simulink model "WEC_Sim_Driver"  (R2013a)
settings: Solver=ode4  StartTime=StartTime  StopTime=EndTime  FixedStep=deltaT  MaxStep=deltaTMax  MinStep=deltaTMin  RelTol=1e-3
undefined symbols (not defined in the file): A_bore, A_c_F, A_c_P, A_rod, angle_arm_aft, Bd, C_aft, deltaT, Gen_Damp, hyd_mot_eff, hydro, hydroForce, Jtot, K_aft, Kd, mooring_c, mooring_k, nonlinear_params, omega_s, p_atm, p_hp, p_lp, pump_vol_eff, r_g, STLfloat, STLplate, Ts, V_hp, V_lp, Vg, X, Y, Z
libraries: nesl_utility x35, sm_lib x14
(part 1 of 2)
settings Model: Creator=cmccomb  LastModifiedBy=sakanne
settings SolverCC: InitialStep=deltaTInitial  MaxConsecutiveZCs=10000  MaxConsecutiveMinStep=20  ZeroCrossAlgorithm=Adaptive
settings DataIOCC: LimitDataPoints=off  SignalLoggingSaveFormat=ModelDataLogs
settings OptimizationCC: ExpressionDepthLimit=2147483647
settings DebuggingCC: FcnCallInpInsideContextMsg=EnableAllAsWarning

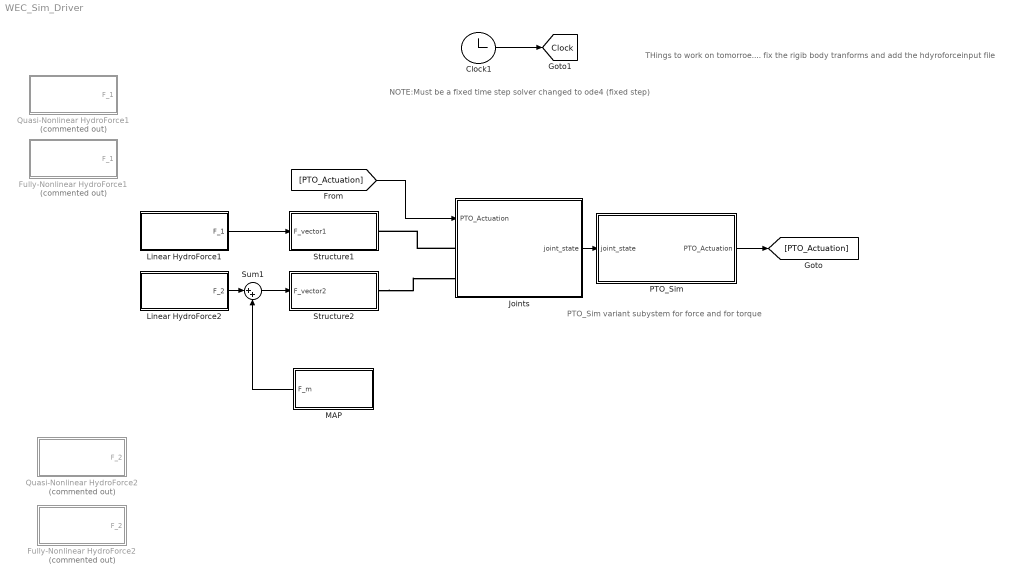
== system WEC_Sim_Driver ==
  note: THings to work on tomorroe....
      | fix the rigib body tranforms and add the hdyroforceinput file
  note: NOTE:Must be a fixed time step solver
      | changed to ode4 (fixed step)
  note: PTO_Sim variant subystem for force and for torque
  Clock1 : Clock
      settings: Decimation=50
  Fully-Nonlinear HydroForce1 : Subsystem  Commented=on  mask{K_mat=hydroForce.HGRes_1, Am_mat=hydroForce.Fadm_1, B_mat=hydroForce.Fdmp_1, X_mat=hydroForce.F_extTime_1}
      mask prompts: K_mat "Stiffness Matrix"; Am_mat "Added Mass Matrix"; B_mat "Radiation Damping Matrix"; X_mat "Excitation Matrix"
  Fully-Nonlinear HydroForce2 : Subsystem  Commented=on  mask{K_mat=hydroForce.HGRes_2, Am_mat=hydroForce.Fadm_2, B_mat=hydroForce.Fdmp_2, X_mat=hydroForce.F_extTime_2}
      mask prompts: K_mat "Stiffness Matrix"; Am_mat "Added Mass Matrix"; B_mat "Radiation Damping Matrix"; X_mat "Excitation Matrix"
  Joints : Subsystem  Variant=on
  Linear HydroForce1 : Subsystem  mask{K_mat=hydroForce.HGRes_1, Am_mat=hydroForce.Fadm_1, B_mat=hydroForce.Fdmp_1, X_mat=hydroForce.F_extTime_1}
      mask prompts: K_mat "Stiffness Matrix"; Am_mat "Added Mass Matrix"; B_mat "Radiation Damping Matrix"; X_mat "Excitation Matrix"
  Linear HydroForce2 : Subsystem  mask{K_mat=hydroForce.HGRes_2, Am_mat=hydroForce.Fadm_2, B_mat=hydroForce.Fdmp_2, X_mat=hydroForce.F_extTime_2}
      mask prompts: K_mat "Stiffness Matrix"; Am_mat "Added Mass Matrix"; B_mat "Radiation Damping Matrix"; X_mat "Excitation Matrix"
  MAP : Subsystem
  PTO_Sim : Subsystem
  Quasi-Nonlinear HydroForce1 : Subsystem  Commented=on  mask{K_mat=hydroForce.HGRes_1, Am_mat=hydroForce.Fadm_1, B_mat=hydroForce.Fdmp_1, X_mat=hydroForce.F_extTime_1}
      mask prompts: K_mat "Stiffness Matrix"; Am_mat "Added Mass Matrix"; B_mat "Radiation Damping Matrix"; X_mat "Excitation Matrix"
  Quasi-Nonlinear HydroForce2 : Subsystem  Commented=on  mask{K_mat=hydroForce.HGRes_2, Am_mat=hydroForce.Fadm_2, B_mat=hydroForce.Fdmp_2, X_mat=hydroForce.F_extTime_2}
      mask prompts: K_mat "Stiffness Matrix"; Am_mat "Added Mass Matrix"; B_mat "Radiation Damping Matrix"; X_mat "Excitation Matrix"
  Structure1 : Subsystem
  Structure2 : Subsystem
  Sum1 : Sum  Inputs=|++
  tag scope: Clock=global
  wires:
  Joints/1(joint_state) -> PTO_Sim/1(joint_state)
  MAP/1(F_m) -> Sum1/2
  PTO_Sim/1(PTO_Actuation) -> [PTO_Actuation]
  [PTO_Actuation] -> Joints/1(PTO_Actuation)
  Sum1/1 -> Structure2/1(F_vector2)
  Clock1/1 -> [Clock]
  Linear HydroForce2/1(F_2) -> Sum1/1
  Linear HydroForce1/1(F_1) -> Structure1/1(F_vector1)
  connections:
  Joints/LConn1 -- Structure1/RConn1
  Structure2/RConn1 -- Joints/LConn2

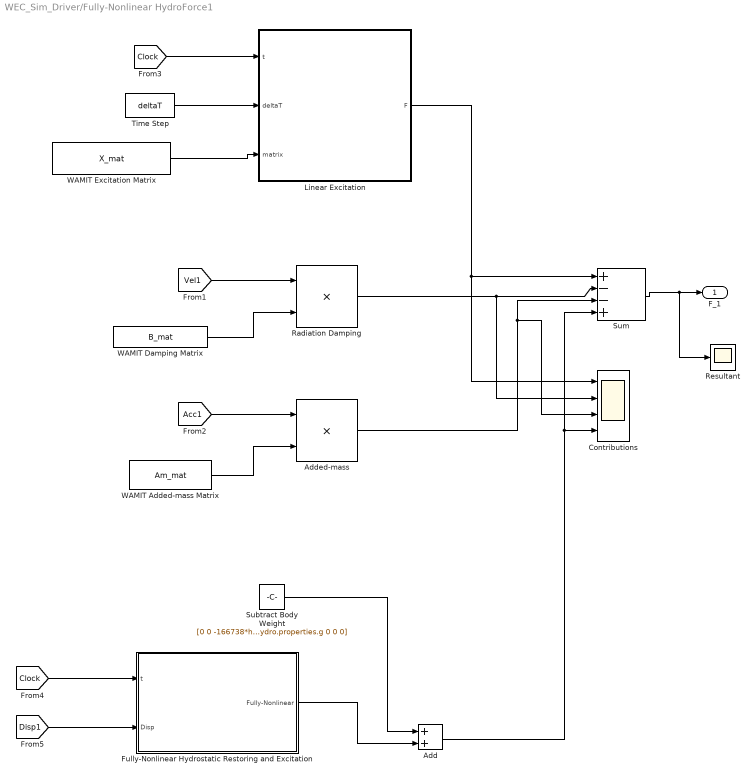
== system WEC_Sim_Driver/Fully-Nonlinear HydroForce1 ==
  Add : Sum
  Added-mass : Product
  Contributions : Scope  NumInputPorts=4
      settings: YMin=-5~-5~-5~-5  YMax=5~5~5~5  SaveName=ScopeData2
  Fully-Nonlinear Hydrostatic Restoring and Excitation : Subsystem  TreatAsAtomicUnit=on
  Linear Excitation : MATLAB Function  TreatAsAtomicUnit=on
  Radiation Damping : Product
  Resultant : Scope
  Subtract Body Weight : Constant  Value=[0 0 -166738*hydro.properties.g 0 0 0]
  Sum : Sum  Inputs=+--+
  Time Step : Constant  Value=deltaT
  WAMIT Added-mass Matrix : Constant  Value=Am_mat  VectorParams1D=off
  WAMIT Damping Matrix : Constant  Value=B_mat  VectorParams1D=off
  WAMIT Excitation Matrix : Constant  Value=X_mat  VectorParams1D=off
  F_1 : Outport
  wires:
  Radiation Damping/1 -> Sum/2, Contributions/2
  [Vel1] -> Radiation Damping/1
  WAMIT Damping Matrix/1 -> Radiation Damping/2
  Added-mass/1 -> Sum/3, Contributions/3
  [Acc1] -> Added-mass/1
  WAMIT Added-mass Matrix/1 -> Added-mass/2
  Sum/1 -> Resultant/1, F_1/1
  [Clock] -> Fully-Nonlinear Hydrostatic Restoring and Excitation/1(t)
  [Disp1] -> Fully-Nonlinear Hydrostatic Restoring and Excitation/2(Disp)
  Subtract Body Weight/1 -> Add/1
  Fully-Nonlinear Hydrostatic Restoring and Excitation/1(Fully-Nonlinear) -> Add/2
  Time Step/1 -> Linear Excitation/2(deltaT)
  WAMIT Excitation Matrix/1 -> Linear Excitation/3(matrix)
  [Clock] -> Linear Excitation/1(t)
  Linear Excitation/1(F) -> Sum/1, Contributions/1
  Add/1 -> Contributions/4, Sum/4

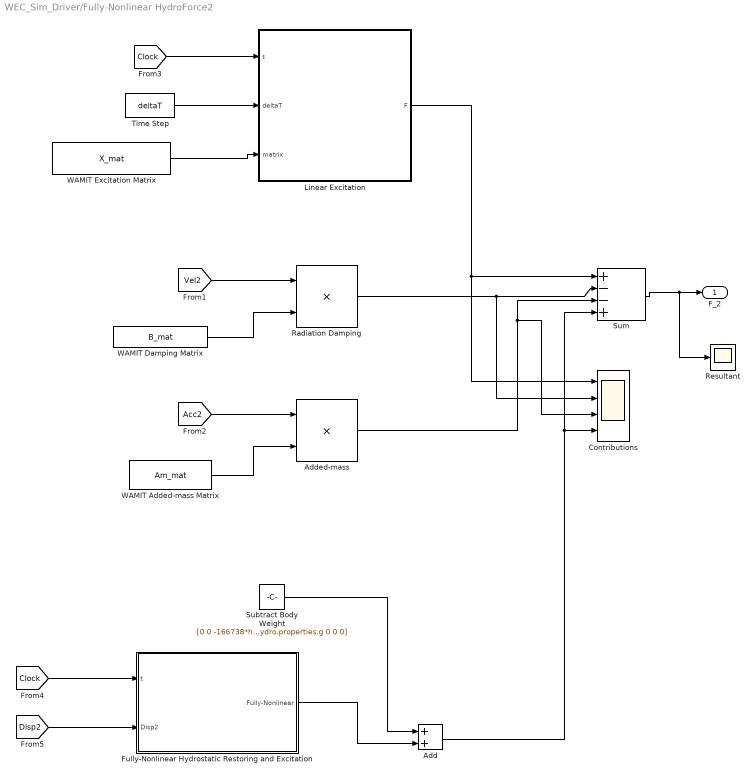
== system WEC_Sim_Driver/Fully-Nonlinear HydroForce2 ==
  Add : Sum
  Added-mass : Product
  Contributions : Scope  NumInputPorts=4
      settings: YMin=-5~-5~-5~-5  YMax=5~5~5~5  SaveName=ScopeData2
  Fully-Nonlinear Hydrostatic Restoring and Excitation : Subsystem  TreatAsAtomicUnit=on
  Linear Excitation : MATLAB Function  TreatAsAtomicUnit=on
  Radiation Damping : Product
  Resultant : Scope
  Subtract Body Weight : Constant  Value=[0 0 -166738*hydro.properties.g 0 0 0]
  Sum : Sum  Inputs=+--+
  Time Step : Constant  Value=deltaT
  WAMIT Added-mass Matrix : Constant  Value=Am_mat  VectorParams1D=off
  WAMIT Damping Matrix : Constant  Value=B_mat  VectorParams1D=off
  WAMIT Excitation Matrix : Constant  Value=X_mat  VectorParams1D=off
  F_2 : Outport
  wires:
  Radiation Damping/1 -> Sum/2, Contributions/2
  [Vel2] -> Radiation Damping/1
  WAMIT Damping Matrix/1 -> Radiation Damping/2
  Added-mass/1 -> Sum/3, Contributions/3
  [Acc2] -> Added-mass/1
  WAMIT Added-mass Matrix/1 -> Added-mass/2
  Sum/1 -> Resultant/1, F_2/1
  [Clock] -> Fully-Nonlinear Hydrostatic Restoring and Excitation/1(t)
  [Disp2] -> Fully-Nonlinear Hydrostatic Restoring and Excitation/2(Disp2)
  Subtract Body Weight/1 -> Add/1
  Fully-Nonlinear Hydrostatic Restoring and Excitation/1(Fully-Nonlinear) -> Add/2
  Time Step/1 -> Linear Excitation/2(deltaT)
  WAMIT Excitation Matrix/1 -> Linear Excitation/3(matrix)
  [Clock] -> Linear Excitation/1(t)
  Linear Excitation/1(F) -> Sum/1, Contributions/1
  Add/1 -> Contributions/4, Sum/4

== system WEC_Sim_Driver/Joints ==
  note: If you have a rotaional joint, you're outputing a torque and must change PTO-Sim to torque model.
      | similar is true to a linear joint and PTO
  note: 1) Only subsystems can be added as variant choices at this level
      | 2) Blocks cannot be connected at this level as connectivity is
      | automatically determined at simulation, based on the active variant
  PTO_Actuation : Inport
  Linear  Joint : Subsystem  VariantControl=VSS_Linear
  Rotational Joint : Subsystem  VariantControl=VSS_Rotation
  Body1 : PMIOPort  Port=1  Side=Left
  Body2 : PMIOPort  Port=2  Side=Left
  joint_state : Outport

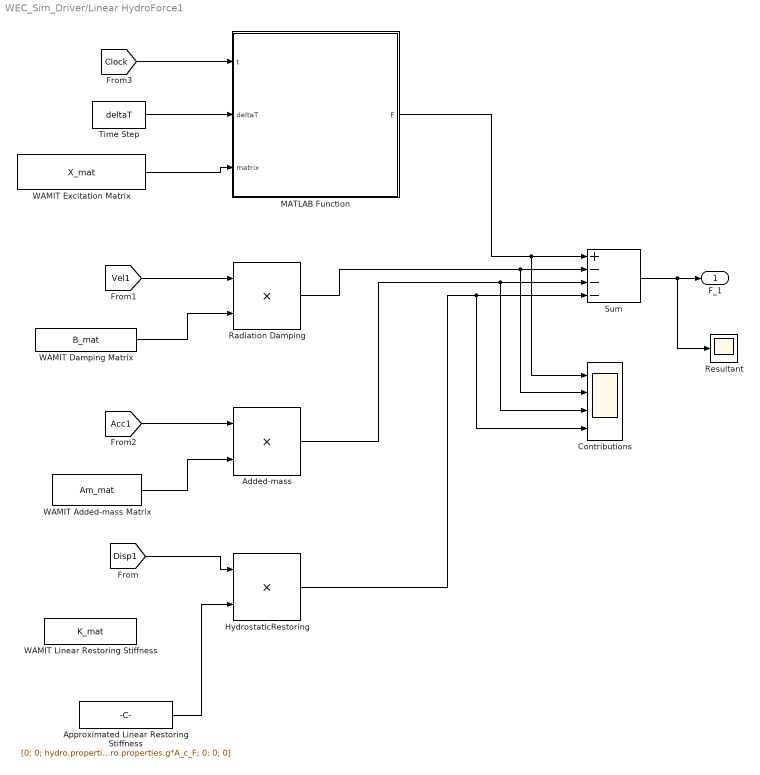
== system WEC_Sim_Driver/Linear HydroForce1 ==
  Added-mass : Product
  Approximated Linear Restoring Stiffness : Constant  Value=[0; 0; hydro.properties.density*hydro.properties.g*A_c_F; 0; 0; 0]  VectorParams1D=off
  Contributions : Scope  NumInputPorts=4
      settings: YMin=-5~-5~-5~-5  YMax=5~5~5~5  SaveName=ScopeData5
  HydrostaticRestoring : Product
  MATLAB Function : MATLAB Function  TreatAsAtomicUnit=on
  Radiation Damping : Product
  Resultant : Scope
      settings: SaveName=ScopeData6
  Sum : Sum  Inputs=+---
  Time Step : Constant  Value=deltaT
  WAMIT Added-mass Matrix : Constant  Value=Am_mat  VectorParams1D=off
  WAMIT Damping Matrix : Constant  Value=B_mat  VectorParams1D=off
  WAMIT Excitation Matrix : Constant  Value=X_mat  VectorParams1D=off
  WAMIT Linear Restoring Stiffness : Constant  Value=K_mat  VectorParams1D=off
  F_1 : Outport
  wires:
  Time Step/1 -> MATLAB Function/2(deltaT)
  WAMIT Excitation Matrix/1 -> MATLAB Function/3(matrix)
  MATLAB Function/1(F) -> Contributions/1, Sum/1
  Sum/1 -> F_1/1, Resultant/1
  WAMIT Added-mass Matrix/1 -> Added-mass/2
  [Acc1] -> Added-mass/1
  Added-mass/1 -> Contributions/3, Sum/3
  [Disp1] -> HydrostaticRestoring/1
  HydrostaticRestoring/1 -> Contributions/4, Sum/4
  WAMIT Damping Matrix/1 -> Radiation Damping/2
  [Vel1] -> Radiation Damping/1
  Radiation Damping/1 -> Contributions/2, Sum/2
  [Clock] -> MATLAB Function/1(t)
  Approximated Linear Restoring Stiffness/1 -> HydrostaticRestoring/2

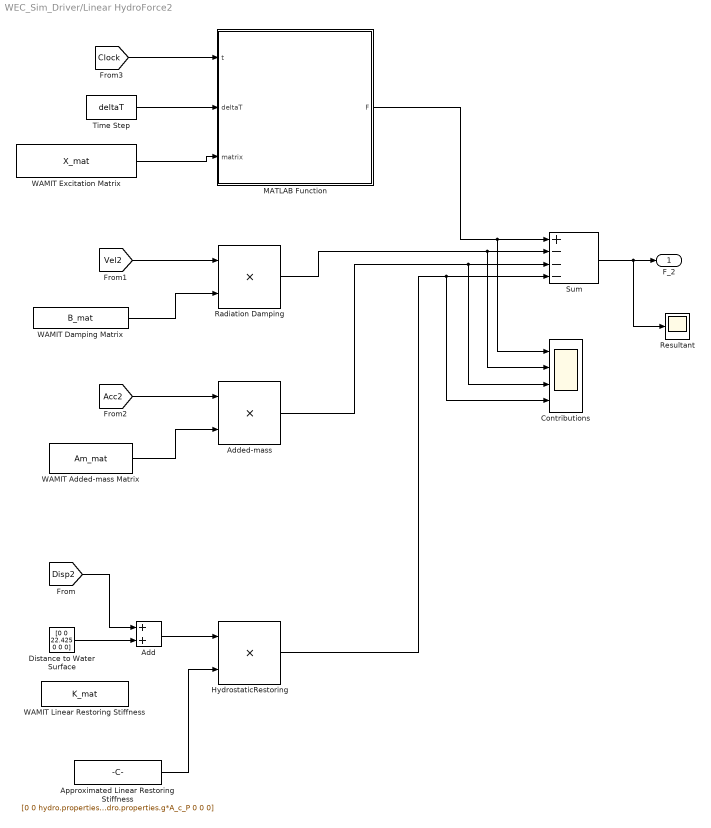
== system WEC_Sim_Driver/Linear HydroForce2 ==
  Add : Sum
  Added-mass : Product
  Approximated Linear Restoring Stiffness : Constant  Value=[0 0 hydro.properties.density*hydro.properties.g*A_c_P 0 0 0]  VectorParams1D=off
  Contributions : Scope  NumInputPorts=4
      settings: YMin=-5~-5~-5~-5  YMax=5~5~5~5  SaveName=ScopeData5
  Distance to Water Surface : Constant  Value=[0 0 22.425 0 0 0]
  HydrostaticRestoring : Product
  MATLAB Function : MATLAB Function  TreatAsAtomicUnit=on
  Radiation Damping : Product
  Resultant : Scope
      settings: SaveName=ScopeData6
  Sum : Sum  Inputs=+---
  Time Step : Constant  Value=deltaT
  WAMIT Added-mass Matrix : Constant  Value=Am_mat  VectorParams1D=off
  WAMIT Damping Matrix : Constant  Value=B_mat  VectorParams1D=off
  WAMIT Excitation Matrix : Constant  Value=X_mat  VectorParams1D=off
  WAMIT Linear Restoring Stiffness : Constant  Value=K_mat  VectorParams1D=off
  F_2 : Outport
  wires:
  Time Step/1 -> MATLAB Function/2(deltaT)
  WAMIT Excitation Matrix/1 -> MATLAB Function/3(matrix)
  MATLAB Function/1(F) -> Contributions/1, Sum/1
  Sum/1 -> F_2/1, Resultant/1
  WAMIT Added-mass Matrix/1 -> Added-mass/2
  [Acc2] -> Added-mass/1
  Added-mass/1 -> Contributions/3, Sum/3
  HydrostaticRestoring/1 -> Contributions/4, Sum/4
  WAMIT Damping Matrix/1 -> Radiation Damping/2
  [Vel2] -> Radiation Damping/1
  Radiation Damping/1 -> Contributions/2, Sum/2
  [Clock] -> MATLAB Function/1(t)
  Approximated Linear Restoring Stiffness/1 -> HydrostaticRestoring/2
  [Disp2] -> Add/1
  Add/1 -> HydrostaticRestoring/1
  Distance to Water Surface/1 -> Add/2

== system WEC_Sim_Driver/MAP ==
  Mooring damping : Gain  Gain=mooring_c  Multiplication=Matrix(K*u)
  Mooring stifness : Gain  Gain=mooring_k  Multiplication=Matrix(K*u)
  sum : Sum  Inputs=--
  F_m : Outport
  wires:
  Mooring stifness/1 -> sum/1
  Mooring damping/1 -> sum/2
  sum/1 -> F_m/1
  [Disp2] -> Mooring stifness/1
  [Vel2] -> Mooring damping/1

== system WEC_Sim_Driver/PTO_Sim ==
  joint_state : Inport
  Drivetrain : Subsystem  Variant=on  VariantControl=Variant
  Electricity_Generation : Subsystem  Variant=on  VariantControl=Variant1
  PTO_Actuation : Outport
  wires:
  Drivetrain/2(omega_Gen) -> Electricity_Generation/1(omega_gen_in)
  Electricity_Generation/1(T_gen_out) -> Drivetrain/2(T_gens_toDrivetrain)
  joint_state/1 -> Drivetrain/1(states_to_Drivetrain)
  Drivetrain/1(T_gen_out) -> PTO_Actuation/1

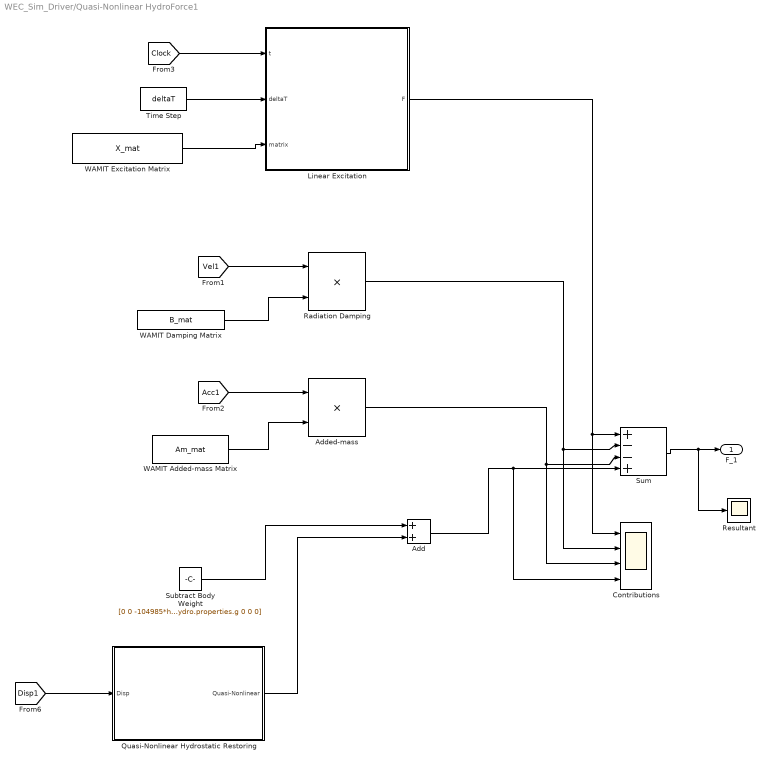
== system WEC_Sim_Driver/Quasi-Nonlinear HydroForce1 ==
  Add : Sum
  Added-mass : Product
  Contributions : Scope  NumInputPorts=4
      settings: YMin=-250000~-900~-35000~-60000  YMax=400000~50~55000~5000  SaveName=ScopeData2
  Linear Excitation : MATLAB Function  TreatAsAtomicUnit=on
  Quasi-Nonlinear Hydrostatic Restoring : Subsystem  TreatAsAtomicUnit=on
  Radiation Damping : Product
  Resultant : Scope
  Subtract Body Weight : Constant  Value=[0 0 -104985*hydro.properties.g 0 0 0]
  Sum : Sum  Inputs=+--+
  Time Step : Constant  Value=deltaT
  WAMIT Added-mass Matrix : Constant  Value=Am_mat  VectorParams1D=off
  WAMIT Damping Matrix : Constant  Value=B_mat  VectorParams1D=off
  WAMIT Excitation Matrix : Constant  Value=X_mat  VectorParams1D=off
  F_1 : Outport
  wires:
  Subtract Body Weight/1 -> Add/1
  Quasi-Nonlinear Hydrostatic Restoring/1(Quasi-Nonlinear) -> Add/2
  Time Step/1 -> Linear Excitation/2(deltaT)
  WAMIT Excitation Matrix/1 -> Linear Excitation/3(matrix)
  [Clock] -> Linear Excitation/1(t)
  [Disp1] -> Quasi-Nonlinear Hydrostatic Restoring/1(Disp)
  Sum/1 -> F_1/1, Resultant/1
  WAMIT Added-mass Matrix/1 -> Added-mass/2
  [Acc1] -> Added-mass/1
  Added-mass/1 -> Contributions/3, Sum/3
  WAMIT Damping Matrix/1 -> Radiation Damping/2
  [Vel1] -> Radiation Damping/1
  Radiation Damping/1 -> Contributions/2, Sum/2
  Linear Excitation/1(F) -> Contributions/1, Sum/1
  Add/1 -> Contributions/4, Sum/4

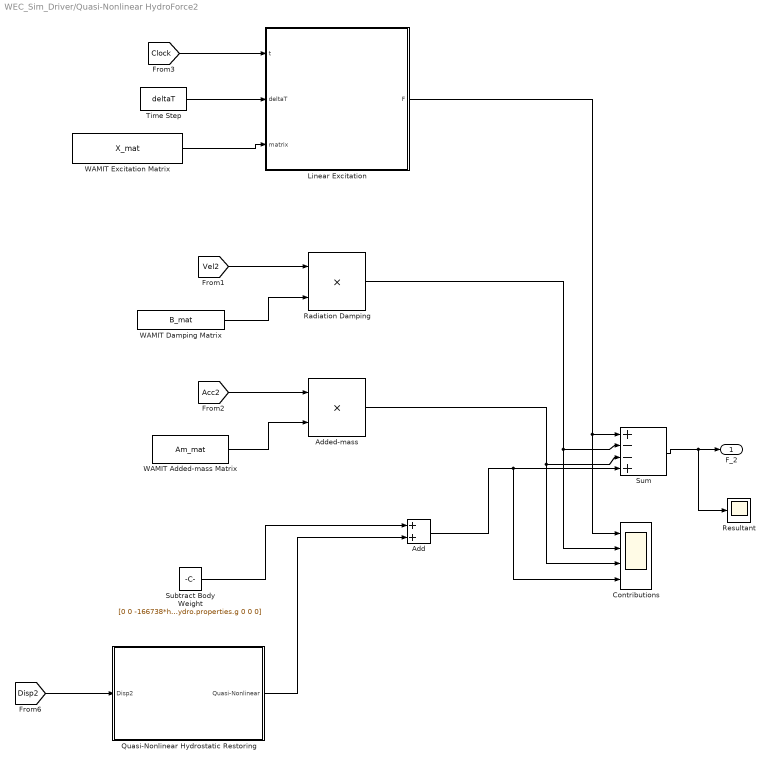
== system WEC_Sim_Driver/Quasi-Nonlinear HydroForce2 ==
  Add : Sum
  Added-mass : Product
  Contributions : Scope  NumInputPorts=4
      settings: YMin=-250000~-900~-35000~-60000  YMax=400000~50~55000~5000  SaveName=ScopeData2
  Linear Excitation : MATLAB Function  TreatAsAtomicUnit=on
  Quasi-Nonlinear Hydrostatic Restoring : Subsystem  TreatAsAtomicUnit=on
  Radiation Damping : Product
  Resultant : Scope
  Subtract Body Weight : Constant  Value=[0 0 -166738*hydro.properties.g 0 0 0]
  Sum : Sum  Inputs=+--+
  Time Step : Constant  Value=deltaT
  WAMIT Added-mass Matrix : Constant  Value=Am_mat  VectorParams1D=off
  WAMIT Damping Matrix : Constant  Value=B_mat  VectorParams1D=off
  WAMIT Excitation Matrix : Constant  Value=X_mat  VectorParams1D=off
  F_2 : Outport
  wires:
  Subtract Body Weight/1 -> Add/1
  Quasi-Nonlinear Hydrostatic Restoring/1(Quasi-Nonlinear) -> Add/2
  Time Step/1 -> Linear Excitation/2(deltaT)
  WAMIT Excitation Matrix/1 -> Linear Excitation/3(matrix)
  [Clock] -> Linear Excitation/1(t)
  [Disp2] -> Quasi-Nonlinear Hydrostatic Restoring/1(Disp2)
  Sum/1 -> F_2/1, Resultant/1
  WAMIT Added-mass Matrix/1 -> Added-mass/2
  [Acc2] -> Added-mass/1
  Added-mass/1 -> Contributions/3, Sum/3
  WAMIT Damping Matrix/1 -> Radiation Damping/2
  [Vel2] -> Radiation Damping/1
  Radiation Damping/1 -> Contributions/2, Sum/2
  Linear Excitation/1(F) -> Contributions/1, Sum/1
  Add/1 -> Contributions/4, Sum/4

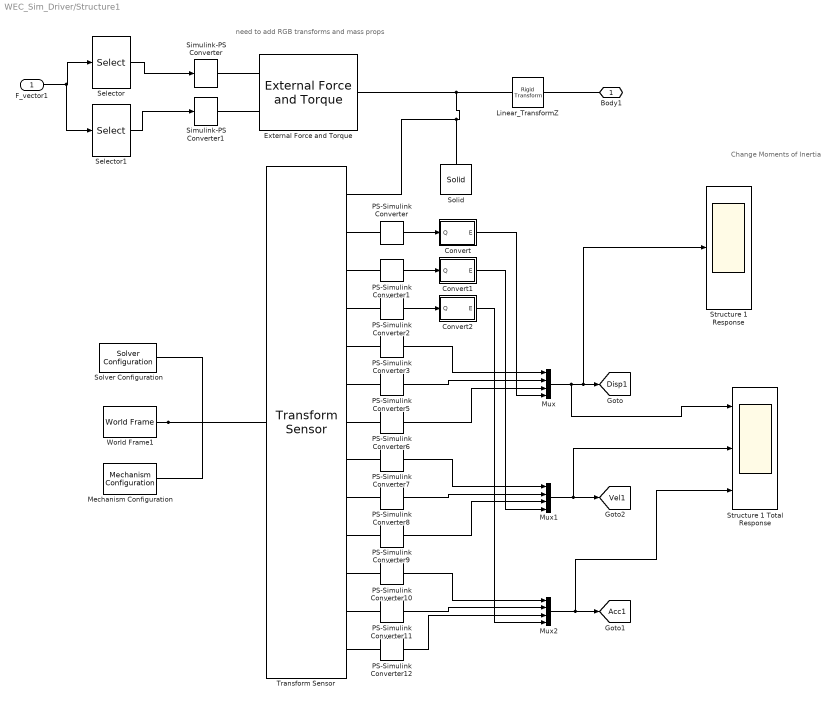
== system WEC_Sim_Driver/Structure1 ==
  note: Change Moments of Inertia
  note: need to add RGB transforms and mass props
  F_vector1 : Inport
  Convert : MATLAB Function  TreatAsAtomicUnit=on
  Convert1 : MATLAB Function  TreatAsAtomicUnit=on
  Convert2 : MATLAB Function  TreatAsAtomicUnit=on
  External Force and Torque : sm_lib/Forces and  Torques/External Force  and Torque  ForceResolutionFrame=AttachedFrame  EnableForceX=off  EnableForceY=off  EnableForceZ=off  EnableForce=on  TorqueResolutionFrame=AttachedFrame  EnableTorqueX=off  EnableTorqueY=off  EnableTorqueZ=off  EnableTorque=on  BlockFunction=simmechanics.library.forces_torques.external_force_torque
  Linear_TransformZ : sm_lib/Frames and  Transforms/Rigid  Transform  TranslationMethod=Cartesian  TranslationLengthUnit=m  TranslationStandardAxis=+Z  TranslationStandardOffset=0  TranslationCartesianOffset=[0 0 -22.425]  TranslationROffset=0  TranslationROffsetUnits=m  TranslationZOffset=0  TranslationZOffsetUnits=m  TranslationThetaOffset=0  TranslationThetaOffsetUnits=deg  RotationMethod=None  RotationAngleUnits=rad  RotationStandardAxis=+Z  RotationAngle=2.0943951023931953  RotationArbitraryAxis=[0.57735026918962584 0.57735026918962584 0.57735026918962584]  FollAlignAxisA=+X  BaseAlignAxisA=+Y  FollAlignAxisB=+Y  BaseAlignAxisB=+Z  BlockFunction=simmechanics.library.frames_transforms.rigid_transform
  Mechanism Configuration : sm_lib/Utilities/Mechanism  Configuration  GravityVector=[0 0 0]  GravityUnits=m/s^2  AllowGravitySignal=off  LinearizationDelta=0.001  BlockFunction=simmechanics.library.utilities.mechanism_configuration
  Mux : Mux
  Mux1 : Mux
  Mux2 : Mux
  PS-Simulink Converter{,1..3,5..12} (12 alike) : nesl_utility/PS-Simulink Converter  PhysicalDomain=network_engine_domain  SubClassName=ps_output  LeftPortType=input  RightPortType=output  PseudoPeriodic=off  Frequencies=[]  Unit=1  AffineConversion=off
  Selector : Selector  InputPortWidth=6  IndexOptions=Index vector (dialog)  Indices=[1:3]  OutputSizes=1
  Selector1 : Selector  InputPortWidth=6  IndexOptions=Index vector (dialog)  Indices=[4:6]  OutputSizes=1
  Simulink-PS Converter : nesl_utility/Simulink-PS Converter  PhysicalDomain=network_engine_domain  SubClassName=ps_input  LeftPortType=input  RightPortType=output  PseudoPeriodic=off  Frequencies=[]  NoiseDistribution=none  NoiseParameters=[]  Unit=1  AffineConversion=off  InputFiltering=off  SimscapeFilterOrder=1  InputFilterTimeConstant=0.001  UdotUserProvided=1
  Simulink-PS Converter1 : nesl_utility/Simulink-PS Converter  PhysicalDomain=network_engine_domain  SubClassName=ps_input  LeftPortType=input  RightPortType=output  PseudoPeriodic=off  Frequencies=[]  NoiseDistribution=none  NoiseParameters=[]  Unit=1  AffineConversion=off  InputFiltering=off  SimscapeFilterOrder=1  InputFilterTimeConstant=0.001  UdotUserProvided=1
  Solid : sm_lib/Body Elements/Solid  InertiaType=Custom  Mass=746000  MassUnits=kg  CenterOfMass=[0 0 0]  CenterOfMassUnits=m  MomentsOfInertia=[913451 913451 1704302]  MomentsOfInertiaUnits=kg*m^2  ProductsOfInertia=[0 0 0]  ProductsOfInertiaUnits=kg*m^2  DensityBased=on  Density=1000  DensityUnits=kg/(m^3)  GraphicType=FromGeometry  MarkerShape=Sphere  MarkerSize=10  MarkerSizeUnits=m  GraphicVisPropType=SimpleVisualProperties  GraphicDiffuseColor=[1 1 1]  GraphicSpecularColor=[0.5 0.5 0.5 1.0]  GraphicAmbientColor=[0.15 0.15 0.15 1.0]  GraphicEmissiveColor=[0.0 0.0 0.0 1.0]  GraphicShininess=75  GraphicOpacity=1  GeometryShape=FromFile  RectangleSize=[1 1]  RectangleSizeUnits=m  BrickDimensions=[1 1 1]  BrickDimensionUnits=m  CylinderRadius=1  CylinderRadiusUnits=m  CylinderLength=1  CylinderLengthUnits=m  SphereRadius=1  SphereRadiusUnits=m  EllipsoidRadii=[1 1 1]  EllipsoidRadiiUnits=m  ExtrusionCrossSection=[1 1; -1 1; -1 -1; 1 -1]  ExtrusionCrossSectionUnits=m  ExtrusionLength=1  ExtrusionLengthUnits=m  PolygonNumSides=3  PolygonOuterRadius=1  PolygonOuterRadiusUnits=m  ExtGeomFileName=\user_inputs\geometry\Float.STL  ExtGeomFileUnits=m  RevolutionCrossSection=[1 1; 1 -1; 2 -1; 2 1]  RevolutionCrossSectionUnits=m  RevolutionExtent=Full  RevolutionAngle=180  RevolutionAngleUnits=deg  BlockFunction=simmechanics.library.body_elements.solid
  Solver Configuration : nesl_utility/Solver Configuration  PhysicalDomain=network_engine_domain  SubClassName=solver  LeftPortType=input  RightPortType=generic  Accelerate=off  Tones=[]  Harmonics=[]  SimulateNoise=off  Profile=off  UseLocalSampling=off  EnableSwitchedLinearOptims=on  FrequencyDomain=off  UseCCode=off  UseNewInitialization=off  DoDC=on  ResidualTolerance=1e-9  UseLocalSolver=off  LocalSolverChoice=NE_BACKWARD_EULER_ADVANCER  LocalSolverSampleTime=.001  DoFixedCost=off  MaxNonlinIter=3  MaxModeIter=2  LinearAlgebra=Sparse  DelaysMemoryBudget=1024
  Structure 1 Response : Scope
      settings: ShowLegends=on  YMin=-1  YMax=1  SaveName=Structure1Response
  Structure 1 Total Response : Scope  NumInputPorts=3
      settings: ShowLegends=on  YMin=-1.5~-0.8~-0.5  YMax=1.5~0.8~0.5  SaveName=ScopeData3
  Transform Sensor : sm_lib/Frames and  Transforms/Transform  Sensor  MeasurementFrame=World  SenseAngle=off  SenseAxis=off  SenseAngle1=off  SenseAngle2=off  SenseAngle3=off  SenseQ=on  SenseR=off  SenseOmegaX=off  SenseOmegaY=off  SenseOmegaZ=off  SenseOmega1=off  SenseOmega2=off  SenseOmega3=off  SenseQDot=on  SenseRDot=off  SenseAlphaX=off  SenseAlphaY=off  SenseAlphaZ=off  SenseAlpha1=off  SenseAlpha2=off  SenseAlpha3=off  SenseQDDot=on  SenseRDDot=off  SenseX=on  SenseY=on  SenseZ=on  SenseRad=off  SenseAzim=off  SenseDist=off  SenseInc=off  SenseXDot=on  SenseYDot=on  SenseZDot=on  SenseRadDot=off  SenseAzimDot=off  SenseDistDot=off  SenseIncDot=off  SenseXDDot=on  SenseYDDot=on  SenseZDDot=on  SenseRadDDot=off  SenseAzimDDot=off  SenseDistDDot=off  SenseIncDDot=off  BlockFunction=simmechanics.library.frames_transforms.transform_sensor
  World Frame1 : sm_lib/Frames and  Transforms/World Frame  BlockFunction=simmechanics.library.frames_transforms.world_frame
  Body1 : PMIOPort  Port=1  Side=Right
  tag scope: Acc1=global, Disp1=global, Vel1=global
  wires:
  Mux/1 -> Structure 1 Total Response/1, Structure 1 Response/1, [Disp1]
  Mux1/1 -> Structure 1 Total Response/2, [Vel1]
  Mux2/1 -> Structure 1 Total Response/3, [Acc1]
  F_vector1/1 -> Selector1/1, Selector/1
  Selector/1 -> Simulink-PS Converter/1
  Selector1/1 -> Simulink-PS Converter1/1
  PS-Simulink Converter2/1 -> Convert2/1(Q)
  PS-Simulink Converter1/1 -> Convert1/1(Q)
  PS-Simulink Converter/1 -> Convert/1(Q)
  Convert/1(E) -> Mux/4
  Convert1/1(E) -> Mux1/4
  Convert2/1(E) -> Mux2/4
  PS-Simulink Converter3/1 -> Mux/1
  PS-Simulink Converter5/1 -> Mux/2
  PS-Simulink Converter6/1 -> Mux/3
  PS-Simulink Converter7/1 -> Mux1/1
  PS-Simulink Converter8/1 -> Mux1/2
  PS-Simulink Converter9/1 -> Mux1/3
  PS-Simulink Converter10/1 -> Mux2/1
  PS-Simulink Converter11/1 -> Mux2/2
  PS-Simulink Converter12/1 -> Mux2/3
  connections:
  Transform Sensor/RConn2 -- PS-Simulink Converter/LConn1
  PS-Simulink Converter1/LConn1 -- Transform Sensor/RConn3
  PS-Simulink Converter2/LConn1 -- Transform Sensor/RConn4
  PS-Simulink Converter3/LConn1 -- Transform Sensor/RConn5
  Transform Sensor/RConn12 -- PS-Simulink Converter11/LConn1
  Transform Sensor/RConn13 -- PS-Simulink Converter12/LConn1
  Transform Sensor/RConn10 -- PS-Simulink Converter9/LConn1
  Transform Sensor/RConn11 -- PS-Simulink Converter10/LConn1
  Transform Sensor/RConn9 -- PS-Simulink Converter8/LConn1
  Transform Sensor/RConn8 -- PS-Simulink Converter7/LConn1
  Transform Sensor/RConn7 -- PS-Simulink Converter6/LConn1
  Transform Sensor/RConn6 -- PS-Simulink Converter5/LConn1
  Simulink-PS Converter/RConn1 -- External Force and Torque/LConn1
  Simulink-PS Converter1/RConn1 -- External Force and Torque/LConn2
  World Frame1/RConn1 -- Solver Configuration/RConn1 -- Transform Sensor/LConn1 -- Mechanism Configuration/RConn1
  External Force and Torque/RConn1 -- Linear_TransformZ/LConn1 -- Solid/RConn1 -- Transform Sensor/RConn1
  Linear_TransformZ/RConn1 -- Body1/RConn1

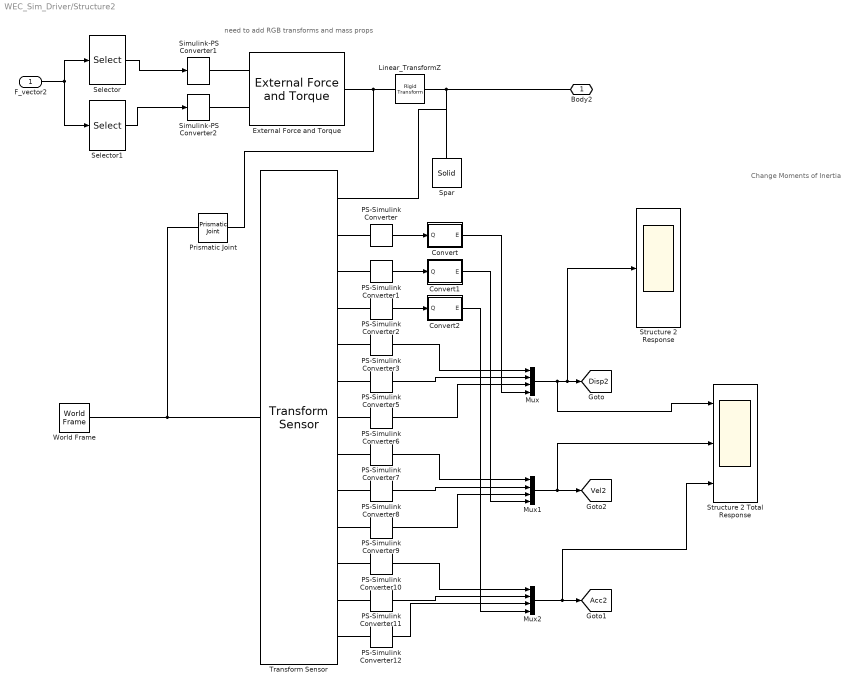
== system WEC_Sim_Driver/Structure2 ==
  note: Change Moments of Inertia
  note: need to add RGB transforms and mass props
  F_vector2 : Inport
  Convert : MATLAB Function  TreatAsAtomicUnit=on
  Convert1 : MATLAB Function  TreatAsAtomicUnit=on
  Convert2 : MATLAB Function  TreatAsAtomicUnit=on
  External Force and Torque : sm_lib/Forces and  Torques/External Force  and Torque  ForceResolutionFrame=AttachedFrame  EnableForceX=off  EnableForceY=off  EnableForceZ=off  EnableForce=on  TorqueResolutionFrame=AttachedFrame  EnableTorqueX=off  EnableTorqueY=off  EnableTorqueZ=off  EnableTorque=on  BlockFunction=simmechanics.library.forces_torques.external_force_torque
  Linear_TransformZ : sm_lib/Frames and  Transforms/Rigid  Transform  TranslationMethod=Cartesian  TranslationLengthUnit=m  TranslationStandardAxis=+Z  TranslationStandardOffset=0  TranslationCartesianOffset=[0 0 22.425]  TranslationROffset=0  TranslationROffsetUnits=m  TranslationZOffset=0  TranslationZOffsetUnits=m  TranslationThetaOffset=0  TranslationThetaOffsetUnits=deg  RotationMethod=None  RotationAngleUnits=rad  RotationStandardAxis=+Z  RotationAngle=2.0943951023931953  RotationArbitraryAxis=[0.57735026918962584 0.57735026918962584 0.57735026918962584]  FollAlignAxisA=+X  BaseAlignAxisA=+Y  FollAlignAxisB=+Y  BaseAlignAxisB=+Z  BlockFunction=simmechanics.library.frames_transforms.rigid_transform
  Mux : Mux
  Mux1 : Mux
  Mux2 : Mux
  PS-Simulink Converter{,1..3,5..12} (12 alike) : nesl_utility/PS-Simulink Converter  PhysicalDomain=network_engine_domain  SubClassName=ps_output  LeftPortType=input  RightPortType=output  PseudoPeriodic=off  Frequencies=[]  Unit=1  AffineConversion=off
  Prismatic Joint : sm_lib/Joints/Prismatic  Joint  SenseConstraintForceX=off  SenseConstraintForceY=off  SenseConstraintForceZ=off  SenseConstraintTorqueX=off  SenseConstraintTorqueY=off  SenseConstraintTorqueZ=off  ConstraintWrenchDir=FollowerOnBase  ConstraintWrenchFrame=BaseFrame  EquilibriumPosition=0  EquilibriumPositionUnits=m  SpringStiffness=0  SpringStiffnessUnits=N/m  DampingCoefficient=0  DampingCoefficientUnits=N/(m/s)  ActuationMode=NoActuation  SensePosition=off  SenseVelocity=off  SenseAcceleration=off  SenseTorqueForce=off  PositionTargetValue=0  PositionTargetValueUnits=m  PositionTargetSpecify=off  PositionTargetPriority=High  VelocityTargetValue=0  VelocityTargetValueUnits=m/s  VelocityTargetSpecify=off  VelocityTargetPriority=High  BlockFunction=simmechanics.library.joints.prismatic_joint
  Selector : Selector  InputPortWidth=6  IndexOptions=Index vector (dialog)  Indices=[1:3]  OutputSizes=1
  Selector1 : Selector  InputPortWidth=6  IndexOptions=Index vector (dialog)  Indices=[4:6]  OutputSizes=1
  Simulink-PS Converter1 : nesl_utility/Simulink-PS Converter  PhysicalDomain=network_engine_domain  SubClassName=ps_input  LeftPortType=input  RightPortType=output  PseudoPeriodic=off  Frequencies=[]  NoiseDistribution=none  NoiseParameters=[]  Unit=1  AffineConversion=off  InputFiltering=off  SimscapeFilterOrder=1  InputFilterTimeConstant=0.001  UdotUserProvided=1
  Simulink-PS Converter2 : nesl_utility/Simulink-PS Converter  PhysicalDomain=network_engine_domain  SubClassName=ps_input  LeftPortType=input  RightPortType=output  PseudoPeriodic=off  Frequencies=[]  NoiseDistribution=none  NoiseParameters=[]  Unit=1  AffineConversion=off  InputFiltering=off  SimscapeFilterOrder=1  InputFilterTimeConstant=0.001  UdotUserProvided=1
  Spar : sm_lib/Body Elements/Solid  InertiaType=Custom  Mass=900000  MassUnits=kg  CenterOfMass=[0 0 0]  CenterOfMassUnits=m  MomentsOfInertia=[15753276 15750563 5053162]  MomentsOfInertiaUnits=kg*m^2  ProductsOfInertia=[1271 13 0]  ProductsOfInertiaUnits=kg*m^2  DensityBased=on  Density=1000  DensityUnits=kg/(m^3)  GraphicType=FromGeometry  MarkerShape=Sphere  MarkerSize=10  MarkerSizeUnits=m  GraphicVisPropType=SimpleVisualProperties  GraphicDiffuseColor=[1 1 1]  GraphicSpecularColor=[0.5 0.5 0.5 1.0]  GraphicAmbientColor=[0.15 0.15 0.15 1.0]  GraphicEmissiveColor=[0.0 0.0 0.0 1.0]  GraphicShininess=75  GraphicOpacity=1  GeometryShape=FromFile  RectangleSize=[1 1]  RectangleSizeUnits=m  BrickDimensions=[1 1 1]  BrickDimensionUnits=m  CylinderRadius=1  CylinderRadiusUnits=m  CylinderLength=1  CylinderLengthUnits=m  SphereRadius=1  SphereRadiusUnits=m  EllipsoidRadii=[1 1 1]  EllipsoidRadiiUnits=m  ExtrusionCrossSection=[1 1; -1 1; -1 -1; 1 -1]  ExtrusionCrossSectionUnits=m  ExtrusionLength=1  ExtrusionLengthUnits=m  PolygonNumSides=3  PolygonOuterRadius=1  PolygonOuterRadiusUnits=m  ExtGeomFileName=\user_inputs\geometry\Plate.STL  ExtGeomFileUnits=m  RevolutionCrossSection=[1 1; 1 -1; 2 -1; 2 1]  RevolutionCrossSectionUnits=m  RevolutionExtent=Full  RevolutionAngle=180  RevolutionAngleUnits=deg  BlockFunction=simmechanics.library.body_elements.solid
  Structure 2 Response : Scope
      settings: ShowLegends=on  YMin=-23  YMax=0  SaveName=Structure2Response
  Structure 2 Total Response : Scope  NumInputPorts=3
      settings: ShowLegends=on  YMin=-0.15~-0.175~-0.1  YMax=0.5~0.175~0.1  SaveName=Structure2Response
  Transform Sensor : sm_lib/Frames and  Transforms/Transform  Sensor  MeasurementFrame=World  SenseAngle=off  SenseAxis=off  SenseAngle1=off  SenseAngle2=off  SenseAngle3=off  SenseQ=on  SenseR=off  SenseOmegaX=off  SenseOmegaY=off  SenseOmegaZ=off  SenseOmega1=off  SenseOmega2=off  SenseOmega3=off  SenseQDot=on  SenseRDot=off  SenseAlphaX=off  SenseAlphaY=off  SenseAlphaZ=off  SenseAlpha1=off  SenseAlpha2=off  SenseAlpha3=off  SenseQDDot=on  SenseRDDot=off  SenseX=on  SenseY=on  SenseZ=on  SenseRad=off  SenseAzim=off  SenseDist=off  SenseInc=off  SenseXDot=on  SenseYDot=on  SenseZDot=on  SenseRadDot=off  SenseAzimDot=off  SenseDistDot=off  SenseIncDot=off  SenseXDDot=on  SenseYDDot=on  SenseZDDot=on  SenseRadDDot=off  SenseAzimDDot=off  SenseDistDDot=off  SenseIncDDot=off  BlockFunction=simmechanics.library.frames_transforms.transform_sensor
  World Frame : sm_lib/Frames and  Transforms/World Frame  BlockFunction=simmechanics.library.frames_transforms.world_frame
  Body2 : PMIOPort  Port=1  Side=Right
  tag scope: Acc2=global, Disp2=global, Vel2=global
  wires:
  F_vector2/1 -> Selector1/1, Selector/1
  Selector/1 -> Simulink-PS Converter1/1
  Selector1/1 -> Simulink-PS Converter2/1
  PS-Simulink Converter2/1 -> Convert2/1(Q)
  PS-Simulink Converter1/1 -> Convert1/1(Q)
  PS-Simulink Converter/1 -> Convert/1(Q)
  Convert/1(E) -> Mux/4
  Convert1/1(E) -> Mux1/4
  Convert2/1(E) -> Mux2/4
  PS-Simulink Converter3/1 -> Mux/1
  PS-Simulink Converter5/1 -> Mux/2
  PS-Simulink Converter6/1 -> Mux/3
  PS-Simulink Converter7/1 -> Mux1/1
  PS-Simulink Converter8/1 -> Mux1/2
  PS-Simulink Converter9/1 -> Mux1/3
  PS-Simulink Converter10/1 -> Mux2/1
  PS-Simulink Converter11/1 -> Mux2/2
  PS-Simulink Converter12/1 -> Mux2/3
  Mux/1 -> Structure 2 Total Response/1, Structure 2 Response/1, [Disp2]
  Mux1/1 -> Structure 2 Total Response/2, [Vel2]
  Mux2/1 -> Structure 2 Total Response/3, [Acc2]
  connections:
  Simulink-PS Converter1/RConn1 -- External Force and Torque/LConn1
  Simulink-PS Converter2/RConn1 -- External Force and Torque/LConn2
  Transform Sensor/RConn9 -- PS-Simulink Converter8/LConn1
  Transform Sensor/RConn13 -- PS-Simulink Converter12/LConn1
  Transform Sensor/RConn11 -- PS-Simulink Converter10/LConn1
  Transform Sensor/RConn7 -- PS-Simulink Converter6/LConn1
  Transform Sensor/RConn6 -- PS-Simulink Converter5/LConn1
  PS-Simulink Converter3/LConn1 -- Transform Sensor/RConn5
  Transform Sensor/RConn12 -- PS-Simulink Converter11/LConn1
  Transform Sensor/RConn8 -- PS-Simulink Converter7/LConn1
  PS-Simulink Converter2/LConn1 -- Transform Sensor/RConn4
  World Frame/RConn1 -- Prismatic Joint/LConn1 -- Transform Sensor/LConn1
  Transform Sensor/RConn2 -- PS-Simulink Converter/LConn1
  Transform Sensor/RConn10 -- PS-Simulink Converter9/LConn1
  PS-Simulink Converter1/LConn1 -- Transform Sensor/RConn3
  Spar/RConn1 -- Transform Sensor/RConn1 -- Body2/RConn1 -- Linear_TransformZ/LConn1
  Prismatic Joint/RConn1 -- Linear_TransformZ/RConn1 -- External Force and Torque/RConn1

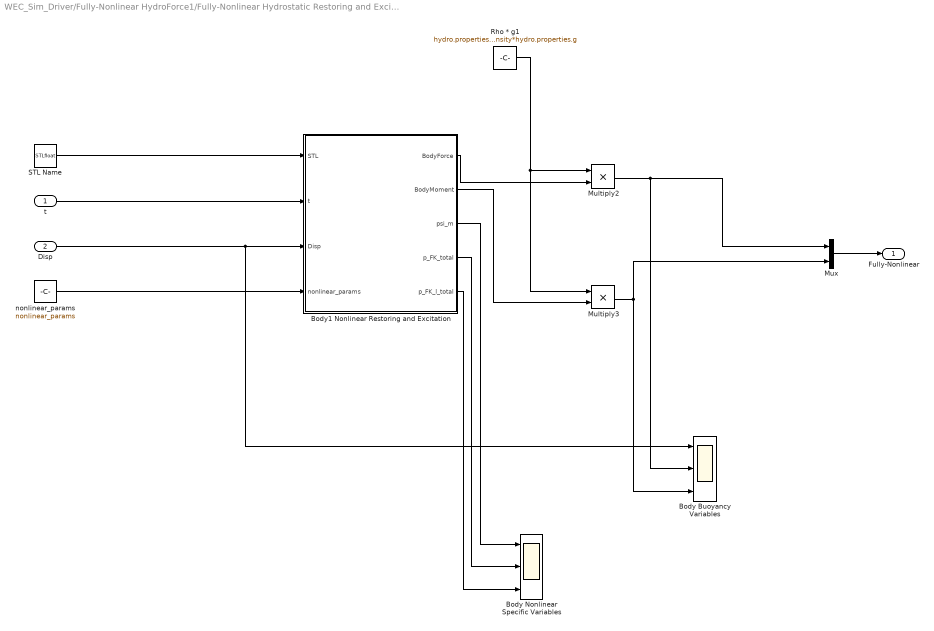
== system WEC_Sim_Driver/Fully-Nonlinear HydroForce1/Fully-Nonlinear Hydrostatic Restoring and Excitation ==
  t : Inport
  Disp : Inport  Port=2
  Body Buoyancy Variables : Scope  NumInputPorts=3
      settings: ShowLegends=on  TimeRange=0.1426953567383918  YMin=-18.5715~0~-0.004  YMax=-16.8027~1500~0.0005  SaveName=AF_buoyancy6
  Body Nonlinear Specific Variables : Scope  NumInputPorts=3
      settings: ShowLegends=on  TimeRange=0.1426953567383918  YMin=-17.6343~0~-0.016  YMax=-17.6337~1500~0  SaveName=spar_nonlinear1
  Body1 Nonlinear Restoring and Excitation : MATLAB Function  TreatAsAtomicUnit=on
  Multiply2 : Product  Inputs=**
  Multiply3 : Product  Inputs=**
  Mux : Mux  Inputs=2
  Rho * g1 : Constant  Value=hydro.properties.density*hydro.properties.g
  STL Name : Constant  Value=STLfloat  VectorParams1D=off
  nonlinear_params : Constant  Value=nonlinear_params  VectorParams1D=off
  Fully-Nonlinear : Outport
  wires:
  Multiply3/1 -> Body Buoyancy Variables/3, Mux/2
  Multiply2/1 -> Body Buoyancy Variables/2, Mux/1
  Body1 Nonlinear Restoring and Excitation/5(p_FK_l_total) -> Body Nonlinear Specific Variables/3
  Body1 Nonlinear Restoring and Excitation/4(p_FK_total) -> Body Nonlinear Specific Variables/2
  Body1 Nonlinear Restoring and Excitation/3(psi_m) -> Body Nonlinear Specific Variables/1
  t/1 -> Body1 Nonlinear Restoring and Excitation/2(t)
  nonlinear_params/1 -> Body1 Nonlinear Restoring and Excitation/4(nonlinear_params)
  Body1 Nonlinear Restoring and Excitation/2(BodyMoment) -> Multiply3/2
  Body1 Nonlinear Restoring and Excitation/1(BodyForce) -> Multiply2/2
  Rho * g1/1 -> Multiply2/1, Multiply3/1
  STL Name/1 -> Body1 Nonlinear Restoring and Excitation/1(STL)
  Mux/1 -> Fully-Nonlinear/1
  Disp/1 -> Body Buoyancy Variables/1, Body1 Nonlinear Restoring and Excitation/3(Disp)

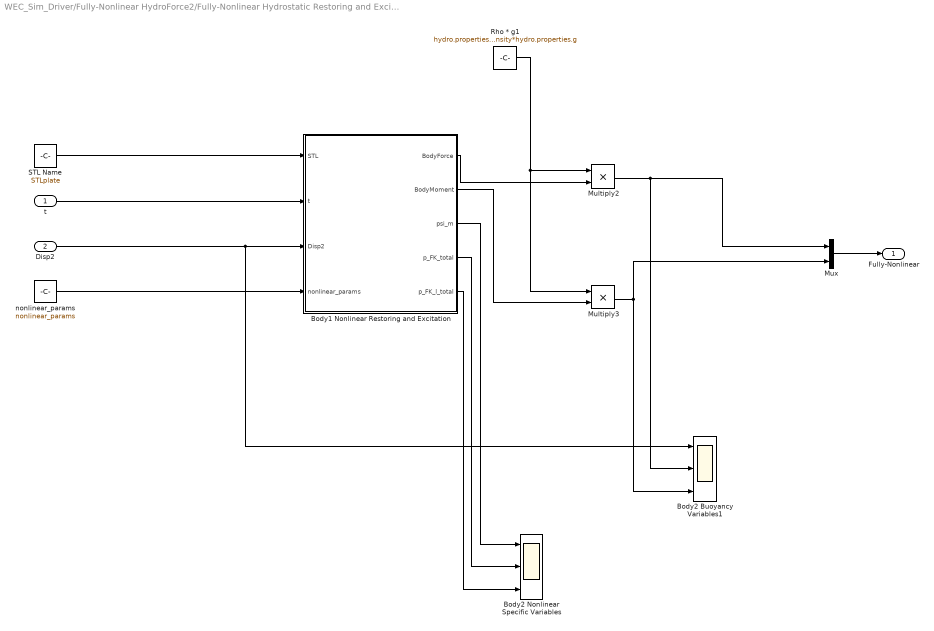
== system WEC_Sim_Driver/Fully-Nonlinear HydroForce2/Fully-Nonlinear Hydrostatic Restoring and Excitation ==
  t : Inport
  Disp2 : Inport  Port=2
  Body1 Nonlinear Restoring and Excitation : MATLAB Function  TreatAsAtomicUnit=on
  Body2 Buoyancy Variables1 : Scope  NumInputPorts=3
      settings: ShowLegends=on  TimeRange=0.1426953567383918  YMin=-18.5715~0~-0.004  YMax=-16.8027~1500~0.0005  SaveName=BodyBuoyancyVars
  Body2 Nonlinear Specific Variables : Scope  NumInputPorts=3
      settings: ShowLegends=on  TimeRange=0.1426953567383918  YMin=-17.6343~0~-0.016  YMax=-17.6337~1500~0  SaveName=NonlinearVars
  Multiply2 : Product  Inputs=**
  Multiply3 : Product  Inputs=**
  Mux : Mux  Inputs=2
  Rho * g1 : Constant  Value=hydro.properties.density*hydro.properties.g
  STL Name : Constant  Value=STLplate  VectorParams1D=off
  nonlinear_params : Constant  Value=nonlinear_params  VectorParams1D=off
  Fully-Nonlinear : Outport
  wires:
  Multiply3/1 -> Body2 Buoyancy Variables1/3, Mux/2
  Multiply2/1 -> Body2 Buoyancy Variables1/2, Mux/1
  Body1 Nonlinear Restoring and Excitation/5(p_FK_l_total) -> Body2 Nonlinear Specific Variables/3
  Body1 Nonlinear Restoring and Excitation/4(p_FK_total) -> Body2 Nonlinear Specific Variables/2
  Body1 Nonlinear Restoring and Excitation/3(psi_m) -> Body2 Nonlinear Specific Variables/1
  t/1 -> Body1 Nonlinear Restoring and Excitation/2(t)
  nonlinear_params/1 -> Body1 Nonlinear Restoring and Excitation/4(nonlinear_params)
  Body1 Nonlinear Restoring and Excitation/2(BodyMoment) -> Multiply3/2
  Body1 Nonlinear Restoring and Excitation/1(BodyForce) -> Multiply2/2
  Rho * g1/1 -> Multiply2/1, Multiply3/1
  STL Name/1 -> Body1 Nonlinear Restoring and Excitation/1(STL)
  Mux/1 -> Fully-Nonlinear/1
  Disp2/1 -> Body2 Buoyancy Variables1/1, Body1 Nonlinear Restoring and Excitation/3(Disp2)

== system WEC_Sim_Driver/Joints/Linear  Joint ==
  note: Prismatic Joints can only be actuated in the z-direction,
      | so if you want to actuate it in a different direction you must use transformations
  PTO_Actuation : Inport
  Mux : Mux  Inputs=2
  PS-Simulink Converter : nesl_utility/PS-Simulink Converter  PhysicalDomain=network_engine_domain  SubClassName=ps_output  LeftPortType=input  RightPortType=output  PseudoPeriodic=off  Frequencies=[]  Unit=1  AffineConversion=off
  PS-Simulink Converter1 : nesl_utility/PS-Simulink Converter  PhysicalDomain=network_engine_domain  SubClassName=ps_output  LeftPortType=input  RightPortType=output  PseudoPeriodic=off  Frequencies=[]  Unit=1  AffineConversion=off
  Prismatic Joint : sm_lib/Joints/Prismatic  Joint  SenseConstraintForceX=off  SenseConstraintForceY=off  SenseConstraintForceZ=off  SenseConstraintTorqueX=off  SenseConstraintTorqueY=off  SenseConstraintTorqueZ=off  ConstraintWrenchDir=FollowerOnBase  ConstraintWrenchFrame=BaseFrame  EquilibriumPosition=0  EquilibriumPositionUnits=m  SpringStiffness=0  SpringStiffnessUnits=N/m  DampingCoefficient=0  DampingCoefficientUnits=N/(m/s)  ActuationMode=TorqueForceActuation  SensePosition=on  SenseVelocity=on  SenseAcceleration=off  SenseTorqueForce=off  PositionTargetValue=0  PositionTargetValueUnits=m  PositionTargetSpecify=off  PositionTargetPriority=High  VelocityTargetValue=0  VelocityTargetValueUnits=m/s  VelocityTargetSpecify=off  VelocityTargetPriority=High  BlockFunction=simmechanics.library.joints.prismatic_joint
  Relative Motion : Scope
      settings: ShowLegends=on  YMin=-1  YMax=0.8  SaveName=RelativeMotion
  Simulink-PS Converter : nesl_utility/Simulink-PS Converter  PhysicalDomain=network_engine_domain  SubClassName=ps_input  LeftPortType=input  RightPortType=output  PseudoPeriodic=off  Frequencies=[]  NoiseDistribution=none  NoiseParameters=[]  Unit=1  AffineConversion=off  InputFiltering=off  SimscapeFilterOrder=1  InputFilterTimeConstant=0.001  UdotUserProvided=1
  Body1 : PMIOPort  Port=1  Side=Left
  Body2 : PMIOPort  Port=2  Side=Left
  joint_state : Outport
  wires:
  Mux/1 -> joint_state/1
  PS-Simulink Converter/1 -> Relative Motion/1, Mux/1
  PTO_Actuation/1 -> Simulink-PS Converter/1
  PS-Simulink Converter1/1 -> Mux/2
  connections:
  PS-Simulink Converter/LConn1 -- Prismatic Joint/RConn2
  Prismatic Joint/RConn3 -- PS-Simulink Converter1/LConn1
  Simulink-PS Converter/RConn1 -- Prismatic Joint/LConn2
  Body2/RConn1 -- Prismatic Joint/LConn1
  Body1/RConn1 -- Prismatic Joint/RConn1

== system WEC_Sim_Driver/Joints/Rotational Joint ==
  note: ang vel
  note: angle
  note: Revolute Joints can only be actuated in the rz-direction,
      | so if you want to actuate it in a different direction you must use transformations
  PTO_Actuation : Inport
  Mux : Mux  Inputs=2
  PS-Simulink Converter : nesl_utility/PS-Simulink Converter  PhysicalDomain=network_engine_domain  SubClassName=ps_output  LeftPortType=input  RightPortType=output  PseudoPeriodic=off  Frequencies=[]  Unit=1  AffineConversion=off
  PS-Simulink Converter1 : nesl_utility/PS-Simulink Converter  PhysicalDomain=network_engine_domain  SubClassName=ps_output  LeftPortType=input  RightPortType=output  PseudoPeriodic=off  Frequencies=[]  Unit=1  AffineConversion=off
  Revolute Joint : sm_lib/Joints/Revolute Joint  SenseConstraintForceX=off  SenseConstraintForceY=off  SenseConstraintForceZ=off  SenseConstraintTorqueX=off  SenseConstraintTorqueY=off  SenseConstraintTorqueZ=off  ConstraintWrenchDir=FollowerOnBase  ConstraintWrenchFrame=BaseFrame  EquilibriumPosition=0  EquilibriumPositionUnits=deg  SpringStiffness=0  SpringStiffnessUnits=N*m/deg  DampingCoefficient=0  DampingCoefficientUnits=N*m/(deg/s)  ActuationMode=TorqueForceActuation  SensePosition=on  SenseVelocity=on  SenseAcceleration=off  SenseTorqueForce=off  PositionTargetValue=0  PositionTargetValueUnits=deg  PositionTargetSpecify=off  PositionTargetPriority=High  VelocityTargetValue=0  VelocityTargetValueUnits=deg/s  VelocityTargetSpecify=off  VelocityTargetPriority=High  BlockFunction=simmechanics.library.joints.revolute_joint
  Simulink-PS Converter : nesl_utility/Simulink-PS Converter  PhysicalDomain=network_engine_domain  SubClassName=ps_input  LeftPortType=input  RightPortType=output  PseudoPeriodic=off  Frequencies=[]  NoiseDistribution=none  NoiseParameters=[]  Unit=1  AffineConversion=off  InputFiltering=off  SimscapeFilterOrder=1  InputFilterTimeConstant=0.001  UdotUserProvided=1
  Body1 : PMIOPort  Port=1  Side=Left
  Body2 : PMIOPort  Port=2  Side=Left
  joint_state : Outport
  wires:
  Mux/1 -> joint_state/1
  PS-Simulink Converter/1 -> Mux/1
  PS-Simulink Converter1/1 -> Mux/2
  PTO_Actuation/1 -> Simulink-PS Converter/1
  connections:
  PS-Simulink Converter1/LConn1 -- Revolute Joint/RConn3
  Body1/RConn1 -- Revolute Joint/LConn1
  Simulink-PS Converter/RConn1 -- Revolute Joint/LConn2
  Body2/RConn1 -- Revolute Joint/RConn1
  Revolute Joint/RConn2 -- PS-Simulink Converter/LConn1

== system WEC_Sim_Driver/PTO_Sim/Drivetrain ==
  note: 1) Only subsystems can be added as variant choices at this level
      | 2) Blocks cannot be connected at this level as connectivity is
      | automatically determined at simulation, based on the active variant
  states_to_Drivetrain : Inport
  T_gens_toDrivetrain : Inport  Port=2
  Direct-Drive : Subsystem  VariantControl=VSS_DD
  Hydraulics : Subsystem  VariantControl=VSS_Hydraulics
  T_gen_out : Outport
  omega_Gen : Outport  Port=2

== system WEC_Sim_Driver/PTO_Sim/Electricity_Generation ==
  note: 1) Only subsystems can be added as variant choices at this level
      | 2) Blocks cannot be connected at this level as connectivity is
      | automatically determined at simulation, based on the active variant
  omega_gen_in : Inport
  Damper : Subsystem  VariantControl=VSS_Damper
  Spring_Damper : Subsystem  VariantControl=VSS_Spring_Damper
  Thev_equiv : Subsystem  VariantControl=VSS_Thev
  T_gen_out : Outport

== system WEC_Sim_Driver/Quasi-Nonlinear HydroForce1/Quasi-Nonlinear Hydrostatic Restoring ==
  Disp : Inport
  Multiply : Product  Inputs=**
  Multiply1 : Product  Inputs=**
  Mux : Mux  Inputs=2
  Rho * g : Constant  Value=hydro.properties.density*hydro.properties.g
  S Buoyancy Variables : Scope  NumInputPorts=3
      settings: ShowLegends=on  TimeRange=0.1426953567383918  YMin=-1.2~-100000~-1700  YMax=0.1~2.1e+06~100  SaveName=AF_buoyancy
  S Buoyancy Variables1 : Scope
      settings: ShowLegends=on  TimeRange=0.1426953567383918  YMin=-100000  YMax=1.7e+06  SaveName=AF_buoyancy1
  STL Name : Constant  Value=STLfloat  VectorParams1D=off
  Submerged Volume : MATLAB Function  TreatAsAtomicUnit=on
  Quasi-Nonlinear : Outport
  wires:
  Mux/1 -> S Buoyancy Variables1/1, Quasi-Nonlinear/1
  Disp/1 -> Submerged Volume/2(Disp), S Buoyancy Variables/1
  STL Name/1 -> Submerged Volume/1(STL)
  Submerged Volume/2(BodyMoment) -> Multiply1/2
  Submerged Volume/1(BodyForce) -> Multiply/2
  Multiply1/1 -> Mux/2, S Buoyancy Variables/3
  Rho * g/1 -> Multiply/1, Multiply1/1
  Multiply/1 -> S Buoyancy Variables/2, Mux/1

== system WEC_Sim_Driver/Quasi-Nonlinear HydroForce2/Quasi-Nonlinear Hydrostatic Restoring ==
  Disp2 : Inport
  Multiply : Product  Inputs=**
  Multiply1 : Product  Inputs=**
  Mux : Mux  Inputs=2
  Rho * g : Constant  Value=hydro.properties.density*hydro.properties.g
  S Buoyancy Variables : Scope  NumInputPorts=3
      settings: ShowLegends=on  TimeRange=0.1426953567383918  YMin=-50~0~-8000  YMax=0~1.7e+06~0  SaveName=AF_buoyancy
  S Buoyancy Variables1 : Scope
      settings: ShowLegends=on  TimeRange=0.1426953567383918  YMin=-100000  YMax=1.7e+06  SaveName=AF_buoyancy1
  STL Name : Constant  Value=STLplate  VectorParams1D=off
  Submerged Volume : MATLAB Function  TreatAsAtomicUnit=on
  Quasi-Nonlinear : Outport
  wires:
  Mux/1 -> S Buoyancy Variables1/1, Quasi-Nonlinear/1
  Disp2/1 -> Submerged Volume/2(Disp2), S Buoyancy Variables/1
  STL Name/1 -> Submerged Volume/1(STL)
  Submerged Volume/2(BodyMoment) -> Multiply1/2
  Submerged Volume/1(BodyForce) -> Multiply/2
  Multiply1/1 -> Mux/2, S Buoyancy Variables/3
  Rho * g/1 -> Multiply/1, Multiply1/1
  Multiply/1 -> S Buoyancy Variables/2, Mux/1

== system WEC_Sim_Driver/PTO_Sim/Drivetrain/Direct-Drive ==
  states_to_Drivetrain : Inport
  T_gens_toDrivetrain : Inport  Port=2
  Add : Sum  Inputs=-+
  Add1 : Sum
  DDr : Gain  Gain=r_g
  Demux2 : Demux  Outputs=2
  GB_damp : Gain  Gain=Bd
  GB_spring : Gain  Gain=Kd
  aDD1 : Gain  Gain=1/r_g
  T_gen_out : Outport
  omega_Gen : Outport  Port=2
  wires:
  states_to_Drivetrain/1 -> Demux2/1  "state_aft"
  T_gens_toDrivetrain/1 -> aDD1/1  "T_gen"
  Demux2/1 -> GB_spring/1  "disp_aft"
  Demux2/2 -> GB_damp/1, DDr/1  "ang_vel"
  DDr/1 -> omega_Gen/1  "omega_gen_aft"
  aDD1/1 -> Add/2
  Add/1 -> T_gen_out/1
  GB_damp/1 -> Add1/2
  GB_spring/1 -> Add1/1
  Add1/1 -> Add/1

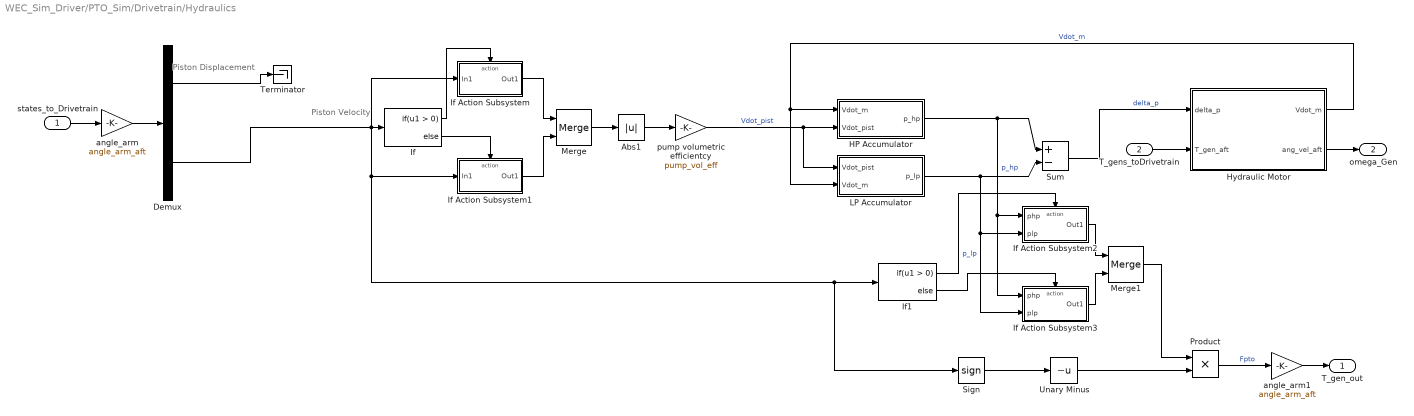
== system WEC_Sim_Driver/PTO_Sim/Drivetrain/Hydraulics ==
  note: Piston Displacement
  note: Piston
      | Velocity
  states_to_Drivetrain : Inport
  T_gens_toDrivetrain : Inport  Port=2
  Abs1 : Abs
  Demux : Demux  Outputs=2
  HP Accumulator : Subsystem
  Hydraulic Motor : Subsystem
  If : If
  If Action Subsystem : Subsystem  TreatAsAtomicUnit=on
  If Action Subsystem1 : Subsystem  TreatAsAtomicUnit=on
  If Action Subsystem2 : Subsystem  TreatAsAtomicUnit=on
  If Action Subsystem3 : Subsystem  TreatAsAtomicUnit=on
  If1 : If
  LP Accumulator : Subsystem
  Merge : Merge
  Merge1 : Merge
  Product : Product  RndMeth=Zero
  Sign : Signum
  Sum : Sum  Inputs=+-
  Terminator : Terminator
  Unary Minus : UnaryMinus
  angle_arm : Gain  Gain=angle_arm_aft
  angle_arm1 : Gain  Gain=angle_arm_aft
  pump volumetric efficientcy : Gain  Gain=pump_vol_eff
  T_gen_out : Outport
  omega_Gen : Outport  Port=2
  wires:
  Demux/2 -> If/1, If Action Subsystem/1(In1), If Action Subsystem1/1(In1), If1/1, Sign/1
  HP Accumulator/1(p_hp) -> Sum/1, If Action Subsystem2/1(php), If Action Subsystem3/1(php)  "p_hp"
  LP Accumulator/1(p_lp) -> Sum/2, If Action Subsystem2/2(plp), If Action Subsystem3/2(plp)  "p_lp"
  Sum/1 -> Hydraulic Motor/1(delta_p)  "delta_p"
  Sign/1 -> Unary Minus/1
  Unary Minus/1 -> Product/2
  Product/1 -> angle_arm1/1  "Fpto"
  Hydraulic Motor/1(Vdot_m) -> LP Accumulator/2(Vdot_m), HP Accumulator/1(Vdot_m)  "Vdot_m"
  If/1 -> If Action Subsystem/Action
  If/2 -> If Action Subsystem1/Action
  pump volumetric efficientcy/1 -> HP Accumulator/2(Vdot_pist), LP Accumulator/1(Vdot_pist)  "Vdot_pist"
  Merge/1 -> Abs1/1
  Abs1/1 -> pump volumetric efficientcy/1
  If1/1 -> If Action Subsystem2/Action
  If1/2 -> If Action Subsystem3/Action
  If Action Subsystem2/1(Out1) -> Merge1/1
  If Action Subsystem3/1(Out1) -> Merge1/2
  If Action Subsystem/1(Out1) -> Merge/1
  If Action Subsystem1/1(Out1) -> Merge/2
  Merge1/1 -> Product/1
  Demux/1 -> Terminator/1
  states_to_Drivetrain/1 -> angle_arm/1
  angle_arm/1 -> Demux/1
  angle_arm1/1 -> T_gen_out/1
  Hydraulic Motor/2(ang_vel_aft) -> omega_Gen/1
  T_gens_toDrivetrain/1 -> Hydraulic Motor/2(T_gen_aft)

== system WEC_Sim_Driver/PTO_Sim/Electricity_Generation/Damper ==
  omega_gen_in : Inport
  Gain : Gain  Gain=Gen_Damp
  Gain1 : Gain  Gain=-1
  T_gen_out : Outport
  wires:
  Gain1/1 -> T_gen_out/1  "T_gen_aft"
  omega_gen_in/1 -> Gain/1
  Gain/1 -> Gain1/1

== system WEC_Sim_Driver/PTO_Sim/Electricity_Generation/Spring_Damper ==
  omega_gen_in : Inport
  Add : Sum  Inputs=--
  Gain : Gain  Gain=C_aft
  Gain1 : Gain  Gain=K_aft
  Integrator : Integrator
  T_gen_out : Outport
  wires:
  Add/1 -> T_gen_out/1  "T_Gen_aft"
  Gain/1 -> Add/2
  Gain1/1 -> Add/1
  omega_gen_in/1 -> Integrator/1, Gain/1
  Integrator/1 -> Gain1/1

== system WEC_Sim_Driver/PTO_Sim/Electricity_Generation/Thev_equiv ==
  omega_gen_in : Inport
  1-D Lookup Table : Lookup_n-D  NumberOfTableDimensions=1  BreakpointsForDimension1=ss  Table=Ts  ExtrapMethod=Clip  UseLastTableValue=on  RndMeth=Simplest  InputSameDT=on
  Constant : Constant  Value=omega_s
  Gain : Gain  Gain=1/omega_s
  Sum : Sum  Inputs=-+
  T_gen_out : Outport
  wires:
  omega_gen_in/1 -> Sum/1  "ang_vel"
  1-D Lookup Table/1 -> T_gen_out/1  "T_gen"
  Sum/1 -> Gain/1
  Gain/1 -> 1-D Lookup Table/1  "Slip_ratio"
  Constant/1 -> Sum/2  "Synch_speed"

== system WEC_Sim_Driver/PTO_Sim/Drivetrain/Hydraulics/HP Accumulator ==
  Vdot_m : Inport
  Vdot_pist : Inport  Port=2
  Constant1 : Constant  Value=p_hp(1)*V_hp(1)^1.4
  Divide : Product  Inputs=*/
  Integrator : Integrator  InitialCondition=V_hp(1)
  Math Function : Math  Operator=pow  SaturateOnIntegerOverflow=on
  Sum1 : Sum  Inputs=+|-
  exponent : Constant  Value=1.4
  p_hp : Outport
  wires:
  Integrator/1 -> Math Function/1
  Divide/1 -> p_hp/1
  Math Function/1 -> Divide/2
  exponent/1 -> Math Function/2
  Constant1/1 -> Divide/1
  Vdot_m/1 -> Sum1/1
  Vdot_pist/1 -> Sum1/2
  Sum1/1 -> Integrator/1

== system WEC_Sim_Driver/PTO_Sim/Drivetrain/Hydraulics/Hydraulic Motor ==
  note: Flow
      | Calculation
  delta_p : Inport
  T_gen_aft : Inport  Port=2
  C : Gain  Gain=Vg/(2*pi*hyd_mot_eff)
  Integrator : Integrator
  Motor Moment of Inertia : Gain  Gain=1/Jtot
  Sum : Sum  Inputs=|+|+|
  Torque Conversion : Gain  Gain=Vg*hyd_mot_eff/(2*pi)
  Vdot_m : Outport
  ang_vel_aft : Outport  Port=2
  wires:
  delta_p/1 -> Torque Conversion/1
  Sum/1 -> Motor Moment of Inertia/1  "Tau_com"
  Motor Moment of Inertia/1 -> Integrator/1  "ang acc"
  Integrator/1 -> ang_vel_aft/1, C/1  "ang_vel"
  Torque Conversion/1 -> Sum/1  "Tau_hm"
  C/1 -> Vdot_m/1
  T_gen_aft/1 -> Sum/2

== system WEC_Sim_Driver/PTO_Sim/Drivetrain/Hydraulics/If Action Subsystem ==
  In1 : Inport
  Action Port : ActionPort
  Gain : Gain  Gain=A_rod
  Out1 : Outport
  wires:
  In1/1 -> Gain/1
  Gain/1 -> Out1/1

== system WEC_Sim_Driver/PTO_Sim/Drivetrain/Hydraulics/If Action Subsystem1 ==
  In1 : Inport
  Action Port : ActionPort
  Gain : Gain  Gain=A_bore
  Out1 : Outport
  wires:
  In1/1 -> Gain/1
  Gain/1 -> Out1/1

== system WEC_Sim_Driver/PTO_Sim/Drivetrain/Hydraulics/If Action Subsystem2 ==
  php : Inport
  plp : Inport  Port=2
  Action Port : ActionPort
  Add : Sum  Inputs=+-
  Gain : Gain  Gain=A_rod
  Gain1 : Gain  Gain=A_bore
  Out1 : Outport
  wires:
  php/1 -> Gain1/1
  plp/1 -> Gain/1
  Gain1/1 -> Add/1
  Gain/1 -> Add/2
  Add/1 -> Out1/1

== system WEC_Sim_Driver/PTO_Sim/Drivetrain/Hydraulics/If Action Subsystem3 ==
  php : Inport
  plp : Inport  Port=2
  Action Port : ActionPort
  Add : Sum  Inputs=+-
  Gain : Gain  Gain=A_bore
  Gain1 : Gain  Gain=A_rod
  Out1 : Outport
  wires:
  php/1 -> Gain1/1
  plp/1 -> Gain/1
  Gain1/1 -> Add/1
  Gain/1 -> Add/2
  Add/1 -> Out1/1

== system WEC_Sim_Driver/PTO_Sim/Drivetrain/Hydraulics/LP Accumulator ==
  Vdot_pist : Inport
  Vdot_m : Inport  Port=2
  Constant2 : Constant  Value=p_lp(1)*V_lp(1)^1.4
  Divide1 : Product  Inputs=*/
  Integrator1 : Integrator  InitialCondition=V_lp(1)
  Math Function1 : Math  Operator=pow  SaturateOnIntegerOverflow=on
  Saturation : Saturate  UpperLimit=inf  LowerLimit=p_atm
  Sum1 : Sum  Inputs=-|+
  exponent2 : Constant  Value=1.4
  p_lp : Outport
  wires:
  Math Function1/1 -> Divide1/2
  exponent2/1 -> Math Function1/2
  Integrator1/1 -> Math Function1/1
  Constant2/1 -> Divide1/1
  Vdot_m/1 -> Sum1/1
  Vdot_pist/1 -> Sum1/2
  Sum1/1 -> Integrator1/1
  Divide1/1 -> Saturation/1
  Saturation/1 -> p_lp/1

== matlab function WEC_Sim_Driver/Structure1/Convert1 ==
  data: Q input; E output
function E  = EulerAngle(Q)
%#codegen
E=zeros(3,1);
E(1) = atan( (2*(Q(1)*Q(2)+Q(3)*Q(4))) / (1-2* (Q(2)^2+Q(3)^2) ) );
E(2) = asin( 2* (Q(1)*Q(3) - Q(4)*Q(2)));
E(3) = atan( (2*(Q(1)*Q(4)+Q(2)*Q(3))) / (1-2* (Q(3)^2+Q(4)^2) ) );

== matlab function WEC_Sim_Driver/Structure1/Convert2 ==
  data: Q input; E output
function E  = EulerAngle(Q)
%#codegen
E=zeros(3,1);
E(1) = atan( (2*(Q(1)*Q(2)+Q(3)*Q(4))) / (1-2* (Q(2)^2+Q(3)^2) ) );
E(2) = asin( 2* (Q(1)*Q(3) - Q(4)*Q(2)));
E(3) = atan( (2*(Q(1)*Q(4)+Q(2)*Q(3))) / (1-2* (Q(3)^2+Q(4)^2) ) );
